simulink model "gravityTestHarness"  (R2024a)
settings: configuration reference "standardSILConfiguraitonParams" (kept outside this file)
settings Model: Creator=jerem  LastModifiedBy=jerem
settings ConfigSetRef: SourceName=standardSILConfiguraitonParams  SourceLocation=Base Workspace

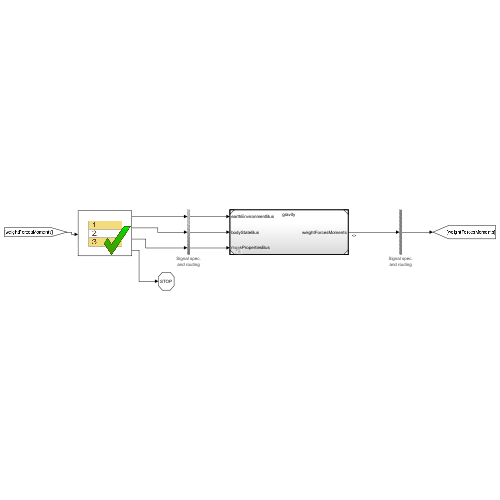
[thumbnail: Simulink's stored preview of the top-level diagram]
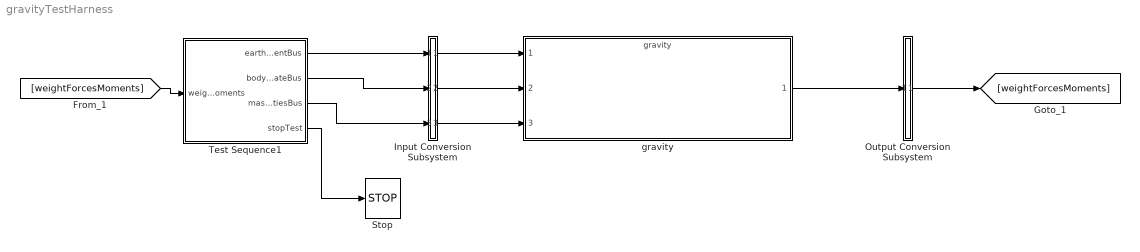
== system gravityTestHarness ==
  Input Conversion Subsystem : Subsystem  Tag=__SLT_ICS__  Description=|
      | Signal spec.
      | and routing
      settings: AttributesFormatString=%<Description>
  Output Conversion Subsystem : Subsystem  Tag=__SLT_OCS__  Description=|
      | Signal spec.
      | and routing
      mask init:
      | ICDictionary = get_param(bdroot, 'DataDictionary');
      | if isempty(ICDictionary)
      |    ICScope = Simulink.data.BaseWorkspace;
      | else
      |    ICScope = Simulink.data.DataDictionary(ICDictionary);
      | end
      | 
      | IC1 = Simulink.Bus.createMATLABStruct('ComponentForcesMomentsBus', [], [1 1], ICScope);
      settings: AttributesFormatString=%<Description>
  Stop : Stop
  Test Sequence1 : Test Sequence  TreatAsAtomicUnit=on
  gravity : ModelReference  ModelNameDialog=gravity  SimulationMode=Normal  ModelReferenceVersion=1.26
  wires:
  Test Sequence1/1(earthEnvironmentBus) -> Input Conversion Subsystem/1(Inport_1)
  Test Sequence1/2(bodyStateBus) -> Input Conversion Subsystem/2(Inport_2)
  Test Sequence1/3(massPropertiesBus) -> Input Conversion Subsystem/3(Inport_3)
  [weightForcesMoments] -> Test Sequence1/1(weightForcesMoments)
  Output Conversion Subsystem/1(Outport_1) -> [weightForcesMoments]
  Test Sequence1/4(stopTest) -> Stop/1
  gravity/1 -> Output Conversion Subsystem/1(Inport_1)
  Input Conversion Subsystem/1(Outport_1) -> gravity/1
  Input Conversion Subsystem/2(Outport_2) -> gravity/2
  Input Conversion Subsystem/3(Outport_3) -> gravity/3

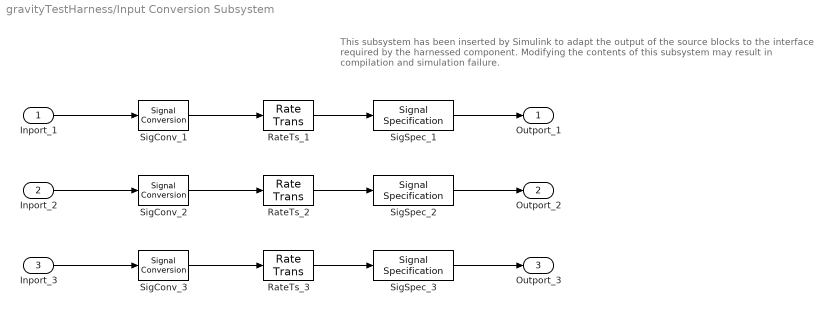
== system gravityTestHarness/Input Conversion Subsystem ==
  note: This subsystem has been inserted by Simulink to adapt the output of the source blocks to the interface required by the harnessed component.
      |  Modifying the contents of this subsystem may result in compilation and simulation failure.
  Inport_1 : Inport
  Inport_2 : Inport  Port=2
  Inport_3 : Inport  Port=3
  RateTs_1 : RateTransition  OutPortSampleTime=0.004
  RateTs_2 : RateTransition  OutPortSampleTime=0.004
  RateTs_3 : RateTransition  OutPortSampleTime=0.004
  SigConv_1 : SignalConversion  ConversionOutput=Virtual bus  OverrideOpt=off
  SigConv_2 : SignalConversion  ConversionOutput=Virtual bus  OverrideOpt=off
  SigConv_3 : SignalConversion  ConversionOutput=Virtual bus  OverrideOpt=off
  SigSpec_1 : SignalSpecification  OutDataTypeStr=Bus: EarthEnvironmentBus  SampleTime=0.004
  SigSpec_2 : SignalSpecification  OutDataTypeStr=Bus: BodyStateBus  SampleTime=0.004
  SigSpec_3 : SignalSpecification  OutDataTypeStr=Bus: MassPropertiesBus  SampleTime=0.004
  Outport_1 : Outport
  Outport_2 : Outport  Port=2
  Outport_3 : Outport  Port=3
  wires:
  SigSpec_1/1 -> Outport_1/1
  RateTs_1/1 -> SigSpec_1/1
  SigConv_1/1 -> RateTs_1/1
  Inport_1/1 -> SigConv_1/1
  SigSpec_2/1 -> Outport_2/1
  RateTs_2/1 -> SigSpec_2/1
  SigConv_2/1 -> RateTs_2/1
  Inport_2/1 -> SigConv_2/1
  SigSpec_3/1 -> Outport_3/1
  RateTs_3/1 -> SigSpec_3/1
  SigConv_3/1 -> RateTs_3/1
  Inport_3/1 -> SigConv_3/1

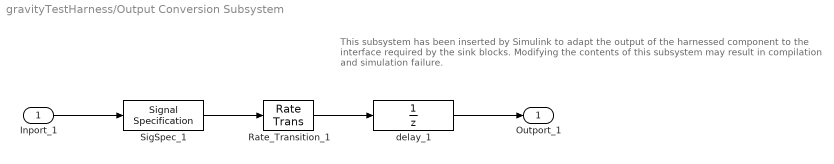
== system gravityTestHarness/Output Conversion Subsystem ==
  note: This subsystem has been inserted by Simulink to adapt the output of the harnessed component to the interface required by the sink blocks.
      |  Modifying the contents of this subsystem may result in compilation and simulation failure.
  Inport_1 : Inport
  Rate_Transition_1 : RateTransition  OutPortSampleTimeOpt=Inherit
  SigSpec_1 : SignalSpecification  OutDataTypeStr=Bus: ComponentForcesMomentsBus  Dimensions=[1]  SampleTime=0.004
  delay_1 : UnitDelay  InitialCondition=IC1  SampleTime=-1
  Outport_1 : Outport
  wires:
  Inport_1/1 -> SigSpec_1/1
  SigSpec_1/1 -> Rate_Transition_1/1
  Rate_Transition_1/1 -> delay_1/1
  delay_1/1 -> Outport_1/1

== stateflow chart gravityTestHarness/Test Sequence1 ==
  state Scenario_1
    state Initialize
      %% Initialize data outputs.
      stopTest = false;
      earthEnvironmentBus.gravityScalar_mps2 = 0;
      bodyStateBus.aircraftVelInNED_mps = zeros(3,1);
      bodyStateBus.aircraftPosInNED_m = zeros(3,1);
      bodyStateBus.aircraftEulerAngles_rad = zeros(3,1);
      bodyStateBus.aircraftVelInBody_mps = zeros(3,1);
      bodyStateBus.aircraftAngVelInBody_radps = zeros(3,1);
      bodyStateBus.aircraftAngAccelInBody_radps2 = zeros(3,1);
      bodyStateBus.aircraftAccelInBody_mps2 = zeros(3,1);
      bodyStateBus.DCM_be = zeros(3,3);
      massPropertiesBus.aircraftMass_kg = 0;
      massPropertiesBus.aircraftCg_m = zeros(3,1);
      massPropertiesBus.aircraftInertiaInBody_kgm2 = zeros(3,3);
    state Define_Test1_Inputs
      % Compute gravity force vector of vehicle aligned with NED frame
      mass_kg = 999;
      gravity_mps2 = 9.81;
      weight_N = mass_kg * gravity_mps2;
      massPropertiesBus.aircraftMass_kg = mass_kg;
      bodyStateBus.DCM_be = eye(3);
      earthEnvironmentBus.gravityScalar_mps2 = gravity_mps2;
    state Test1
      verify(isClose(weightForcesMoments.forcesInBody_N(1), 0));
      verify(isClose(weightForcesMoments.forcesInBody_N(2), 0));
      verify(isClose(weightForcesMoments.forcesInBody_N(3), weight_N));
      verify(isClose(sum(weightForcesMoments.momentsInBody_Nm(1:3)), 0));
    state Define_Test2_Inputs
      % Compute gravity force vector when vehicle is pitched upwards
      pitch_rad = 30*pi/180
      DCM_be =  [cos(pitch_rad) 0 -sin(pitch_rad);
      0 1 0;
      sin(pitch_rad) 0 cos(pitch_rad)];
      massPropertiesBus.aircraftMass_kg = mass_kg;
      bodyStateBus.DCM_be = DCM_be
      earthEnvironmentBus.gravityScalar_mps2 = gravity_mps2;
    state Test2
      verify(isClose(weightForcesMoments.forcesInBody_N(1), -weight_N * sin(pitch_rad)));
      verify(isClose(weightForcesMoments.forcesInBody_N(2), 0));
      verify(isClose(weightForcesMoments.forcesInBody_N(3), weight_N * cos(pitch_rad)));
      verify(isClose(sum(weightForcesMoments.momentsInBody_Nm(1:3)), 0));
    state Define_Test3_Inputs
      % Compute gravity force vector when vehicle is pitched, rolled, and yawed
      yaw_rad = 20*pi/180;
      pitch_rad = 30*pi/180;
      roll_rad = -10*pi/180;
      Rx = [1 0 0;
      0 cos(roll_rad) sin(roll_rad);
      0 -sin(roll_rad) cos(roll_rad)];
      Ry =  [cos(pitch_rad) 0 -sin(pitch_rad);
      0 1 0;
      sin(pitch_rad) 0 cos(pitch_rad)];
      Rz = [cos(yaw_rad) sin(yaw_rad) 0;
      -sin(yaw_rad) cos(yaw_rad) 0;
      0 0 1];
      DCM_be = Rx*Ry*Rz
      massPropertiesBus.aircraftMass_kg = mass_kg;
      bodyStateBus.DCM_be = DCM_be
      earthEnvironmentBus.gravityScalar_mps2= gravity_mps2;
    state Test3
      verify(isClose(weightForcesMoments.forcesInBody_N(1), -weight_N * sin(pitch_rad)));
      verify(isClose(weightForcesMoments.forcesInBody_N(2), weight_N * sin(roll_rad) * cos(pitch_rad)));
      verify(isClose(weightForcesMoments.forcesInBody_N(3), weight_N * cos(roll_rad) * cos(pitch_rad)));
      verify(isClose(sum(weightForcesMoments.momentsInBody_Nm(1:3)), 0));
    state EndTest
      stopTest = true;
    (default) -> Initialize
    Initialize -> Define_Test1_Inputs : [
        | true
        | ]
    Define_Test1_Inputs -> Test1 : [
        | true
        | ]
    Test1 -> Define_Test2_Inputs : [
        | true
        | ]
    Define_Test2_Inputs -> Test2 : [
        | true
        | ]
    Test2 -> Define_Test3_Inputs : [
        | true
        | ]
    Define_Test3_Inputs -> Test3 : [
        | true
        | ]
    Test3 -> EndTest : [
        | true
        | ]
  (default) -> Scenario_1 : {assert(Active_Scenario_Index == 1,'The value of Scenario Parameter ''Active_Scenario_Index'' is not valid. Use the index of the scenario to specify it.')}
  data: weightForcesMoments input Bus: ComponentForcesMomentsBus size=[1]; earthEnvironmentBus output Bus: EarthEnvironmentBus size=[1]; bodyStateBus output Bus: BodyStateBus size=[1]; massPropertiesBus output Bus: MassPropertiesBus size=[1]; Active_Scenario_Index parameter =1; mass_kg local; gravity_mps2 local; weight_N local; pitch_rad local; DCM_be local; yaw_rad local; roll_rad local; Rx local; Ry local; Rz local; stopTest output
